simulink model "serie_tf"  (R2019a)
settings: Solver=VariableStepAuto  StartTime=0.0  StopTime=10.0  RelTol=1e-3
undefined symbols (not defined in the file): Bm, J, LAA, LAF, LFF, ra, rf, Tl, Va, Vf
settings Model: Creator=azizi  LastModifiedBy=azizi

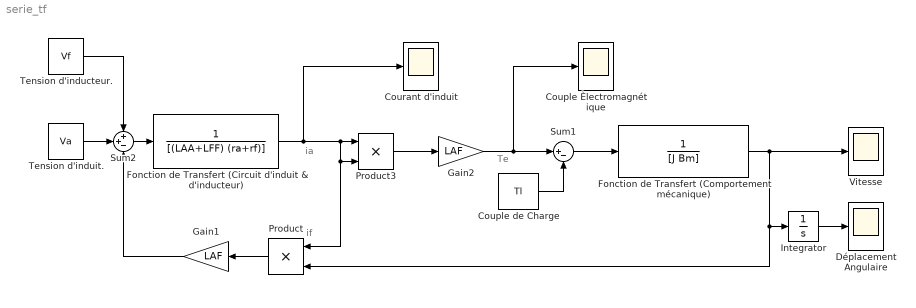
== system serie_tf ==
  note: Te
  note: ia
  note: if
  "Couple de Charge " : Constant  Value=Tl
  Couple Èlectromagnétique : Scope
  Courant d'induit : Scope
  Déplacement Angulaire : Scope
  Fonction de Transfert (Circuit d'induit & d'inducteur) : TransferFcn  Denominator=[(LAA+LFF) (ra+rf)]
  Fonction de Transfert (Comportement mécanique) : TransferFcn  Denominator=[J Bm]
  Gain1 : Gain  Gain=LAF
  Gain2 : Gain  Gain=LAF
  Integrator : Integrator
  Product : Product
  Product3 : Product
  Sum1 : Sum  Inputs=|+-
  Sum2 : Sum  Inputs=++-
  "Tension d'inducteur. " : Constant  Value=Vf
  "Tension d'induit. " : Constant  Value=Va
  Vitesse : Scope
  wires:
  Sum2/1 -> Fonction de Transfert (Circuit d'induit & d'inducteur)/1
  Fonction de Transfert (Circuit d'induit & d'inducteur)/1 -> Courant d'induit/1, Product3/1, Product3/2, Product/1
  Product/1 -> Gain1/1
  Product3/1 -> Gain2/1
  Gain2/1 -> Couple Èlectromagnétique/1, Sum1/1
  Sum1/1 -> Fonction de Transfert (Comportement mécanique)/1
  Fonction de Transfert (Comportement mécanique)/1 -> Vitesse/1, Integrator/1, Product/2
  "Couple de Charge "/1 -> Sum1/2
  Integrator/1 -> Déplacement Angulaire/1
  "Tension d'inducteur. "/1 -> Sum2/1
  "Tension d'induit. "/1 -> Sum2/2
  Gain1/1 -> Sum2/3
